simulink model "Test_N8"  (R2020b)
settings: Solver=ode3  StartTime=0.0  StopTime=inf  FixedStep=0.05  RelTol=1e-3
libraries: XBotBlockToolbox x2, Utilities x1

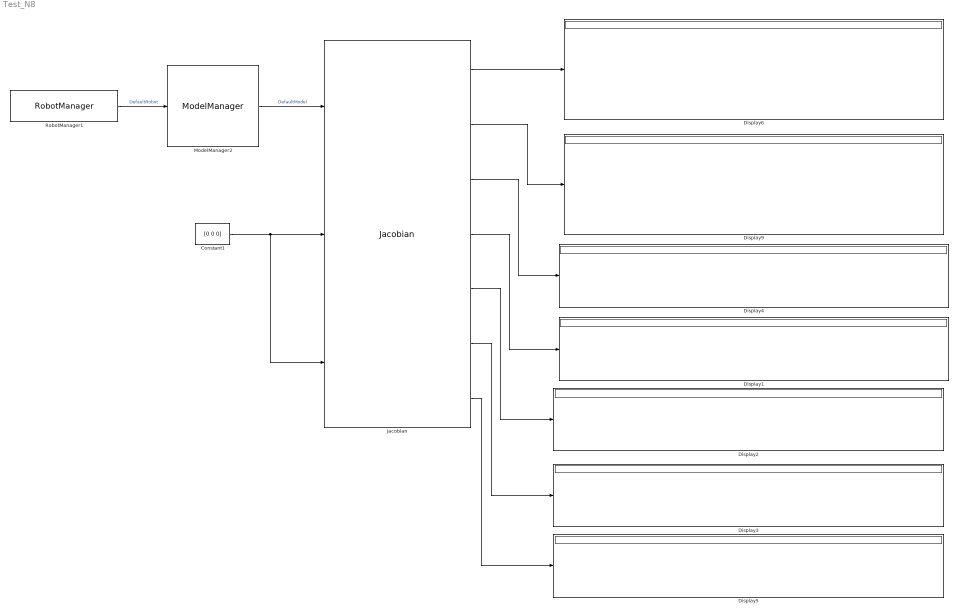
== system Test_N8 ==
  Constant1 : Constant  Value=[0 0 0]
  Display{1..6,9} (7 alike) : Display
  Jacobian : Utilities/Jacobian  ModelName=DefaultModel  JacobianList={ 'J', 'J_postural', 'J_relative', 'J_COM', 'dJcomQdot', 'JdotQdot', 'JdotQdot_relative' }  LinkName=LWrMot3  TargetFrame=LWrMot2  ExternalRef=On  TargetLink=LWrMot3  BaseLink=LWrMot2
  ModelManager2 : XBotBlockToolbox/ModelManager  ModelName=DefaultModel  RobotName=DefaultRobot  UseExtModel=Off  SyncWithRobot=On  GetFloatingBaseList={}  SetFloatingBaseComponent=Off  GravityRequest=Off  ReadingsList={}  MechanicalLimitsList={}  MechanicalLimitsCheck=Off  MechanicalLimitsEnforce=Off  SensorList={}  ReferencesList={}  OldModelName=DefaultModel
  RobotManager1 : XBotBlockToolbox/RobotManager  RobotName=DefaultRobot  ModelName=DefaultModel  UseExtRobot=Off  SyncWithModel=Off  ReadingsList={}  MechanicalLimitsList={}  MechanicalLimitsCheck=Off  MechanicalLimitsEnforce=Off  SensorList={}  ReferencesList={}  OldRobotName=DefaultRobot
  wires:
  RobotManager1/1 -> ModelManager2/1  "DefaultRobot"
  ModelManager2/1 -> Jacobian/1  "DefaultModel"
  Jacobian/2 -> Display9/1
  Jacobian/3 -> Display4/1
  Jacobian/4 -> Display1/1
  Jacobian/5 -> Display2/1
  Jacobian/6 -> Display3/1
  Jacobian/7 -> Display5/1
  Constant1/1 -> Jacobian/3, Jacobian/2
  Jacobian/1 -> Display6/1
